simulink model "multelevel"  (R2017a)
settings: Solver=VariableStepAuto  StartTime=0.0  StopTime=0.5  MaxStep=1e-4  RelTol=1e-3
libraries: powerlib x22, powerlib_meascontrol x2
settings Model: Creator=lenovo 520  LastModifiedBy=lenovo 520

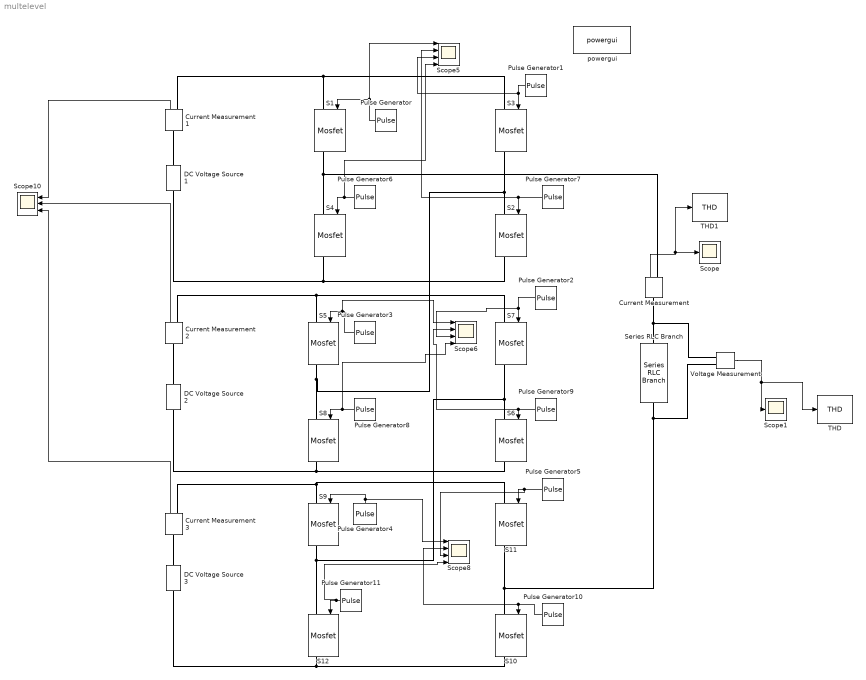
== system multelevel ==
  Current Measurement{,1..3} (4 alike) : powerlib/Measurements/Current Measurement  PhasorSimulation=off  OutputType=Complex  PSBequivalent=0
  DC Voltage Source 1 : powerlib/Electrical Sources/DC Voltage Source  Amplitude=200/3  Measurements=None
  DC Voltage Source 2 : powerlib/Electrical Sources/DC Voltage Source  Amplitude=200/3  Measurements=None
  DC Voltage Source 3 : powerlib/Electrical Sources/DC Voltage Source  Amplitude=200/3  Measurements=None
  Pulse Generator : DiscretePulseGenerator  PulseType=Time based  Period=0.02  PulseWidth=50  PhaseDelay=4.9965e-3
  Pulse Generator1 : DiscretePulseGenerator  PulseType=Time based  Period=0.02  PulseWidth=50  PhaseDelay=0.01-4.9965e-3
  Pulse Generator10 : DiscretePulseGenerator  PulseType=Time based  Period=0.02  PulseWidth=50  PhaseDelay=0.02-6.659e-4
  Pulse Generator11 : DiscretePulseGenerator  PulseType=Time based  Period=0.02  PulseWidth=50  PhaseDelay=0.01+6.659e-4
  Pulse Generator2 : DiscretePulseGenerator  PulseType=Time based  Period=0.02  PulseWidth=50  PhaseDelay=0.01- 2.66e-3
  Pulse Generator3 : DiscretePulseGenerator  PulseType=Time based  Period=0.02  PulseWidth=50  PhaseDelay=2.66e-3
  Pulse Generator4 : DiscretePulseGenerator  PulseType=Time based  Period=0.02  PulseWidth=50  PhaseDelay=6.659e-4
  Pulse Generator5 : DiscretePulseGenerator  PulseType=Time based  Period=0.02  PulseWidth=50  PhaseDelay=0.01-6.659e-4
  Pulse Generator6 : DiscretePulseGenerator  PulseType=Time based  Period=0.02  PulseWidth=50  PhaseDelay=0.01+4.9965e-3
  Pulse Generator7 : DiscretePulseGenerator  PulseType=Time based  Period=0.02  PulseWidth=50  PhaseDelay=0.02-4.9965e-3
  Pulse Generator8 : DiscretePulseGenerator  PulseType=Time based  Period=0.02  PulseWidth=50  PhaseDelay=0.01+ 2.66e-3
  Pulse Generator9 : DiscretePulseGenerator  PulseType=Time based  Period=0.02  PulseWidth=50  PhaseDelay=0.02- 2.66e-3
  S{1..12} (12 alike) : powerlib/Power Electronics/Mosfet  Ron=0  Lon=0  Rd=0  Vfd=0  IC=0  Rs=1e5  Cs=inf  Measurements=on
  Scope : Scope
  Scope1 : Scope
  Scope10 : Scope  NumInputPorts=3
  Scope5 : Scope  NumInputPorts=4
  Scope6 : Scope  NumInputPorts=4
  Scope8 : Scope  NumInputPorts=4
  "Series RLC Branch " : powerlib/Elements/Series RLC Branch  LConnTagsString=__new0  RConnTagsString=__new0  BranchType=RLC  Resistance=1  Inductance=5e-3  SetiL0=off  InitialCurrent=0  Capacitance=0  Setx0=off  InitialVoltage=0  Measurements=None
  THD : powerlib_meascontrol/Measurements/THD  Freq=60  Ts=0
  THD1 : powerlib_meascontrol/Measurements/THD  Freq=60  Ts=0
  Voltage Measurement : powerlib/Measurements/Voltage Measurement  PhasorSimulation=off  OutputType=Complex  PSBequivalent=0
  powergui : powerlib/powergui  Priority=1  SimulationMode=Continuous  SampleTime=50e-6  frequency=60  Iterations=50  frequencyindice=0  Pbase=100e6  ErrMax=1e-4  UnitsV=kV  UnitsW=MW  buscounter=0  FunctionMessages=off  echomessages=off  EnableUseOfTLC=off  CurrentSourceSwitches=off  DisableSnubberDevices=off  DisableRonSwitches=off  DisableVfSwitches=off  DisplayEquations=off  SolverType=Tustin/Backward Euler (TBE)  Interpol=off  ExternalGateDelay=off  methode=off  Ts=100  x0status=blocks  SPID=on  SwTol=0  HookPort=off  RestoreLinks=warning  ResistiveCurrentMeasurement=off  Frange=[0:2:500]  Ylog=off  Xlog=on  ShowGrid=off  save=off  variable=ZData  structure=voltout  ZoomFFT=off  StartTime=0.08  cycles=10  DisplayStyle=1  fundamental=50  FreqAxis=off  MaxFrequency=500  frequencyindicesteady=1  RmsSteady=1  display=off
  wires:
  Pulse Generator/1 -> Scope5/1, S1/1
  Pulse Generator1/1 -> Scope5/3, S3/1
  Pulse Generator4/1 -> S9/1, Scope8/1
  Pulse Generator5/1 -> Scope8/3, S11/1
  Current Measurement/1 -> Scope/1, THD1/1
  Voltage Measurement/1 -> THD/1, Scope1/1
  Current Measurement2/1 -> Scope10/2
  Current Measurement3/1 -> Scope10/3
  Current Measurement1/1 -> Scope10/1
  Pulse Generator6/1 -> Scope5/4, S4/1
  Pulse Generator7/1 -> Scope5/2, S2/1
  Pulse Generator3/1 -> Scope6/1, S5/1
  Pulse Generator2/1 -> Scope6/3, S7/1
  Pulse Generator8/1 -> Scope6/4, S8/1
  Pulse Generator9/1 -> Scope6/2, S6/1
  Pulse Generator10/1 -> Scope8/2, S10/1
  Pulse Generator11/1 -> Scope8/4, S12/1
  connections:
  S3/LConn1 -- Current Measurement1/RConn1 -- S1/LConn1
  S1/RConn1 -- Current Measurement/RConn1 -- S4/LConn1
  S4/RConn1 -- DC Voltage Source 1/LConn1 -- S2/RConn1
  S7/LConn1 -- Current Measurement2/RConn1 -- S5/LConn1
  S5/RConn1 -- S8/LConn1 -- S3/RConn1 -- S2/LConn1
  S8/RConn1 -- S6/RConn1 -- DC Voltage Source 2/LConn1
  S11/LConn1 -- Current Measurement3/RConn1 -- S9/LConn1
  S9/RConn1 -- S12/LConn1 -- S6/LConn1 -- S7/RConn1
  S11/RConn1 -- Voltage Measurement/LConn2 -- "Series RLC Branch "/RConn1 -- S10/LConn1
  DC Voltage Source 3/LConn1 -- S10/RConn1 -- S12/RConn1
  Current Measurement1/LConn1 -- DC Voltage Source 1/RConn1
  Current Measurement2/LConn1 -- DC Voltage Source 2/RConn1
  Current Measurement3/LConn1 -- DC Voltage Source 3/RConn1
  "Series RLC Branch "/LConn1 -- Current Measurement/LConn1 -- Voltage Measurement/LConn1
